simulink library "courseFollow_cl"  (R2018b)
settings: Solver=VariableStepAuto  StartTime=0.0  StopTime=10.0  RelTol=1e-3
values from neighbouring files (symbols this model uses):
  a = parseLogsout    [courseFollow_plant_ts.m]    (also in testUntilRoll_ts.m)
libraries: vectorNormalizer_ul x3, schmehlTangentRotation_ul x1, angleBtw2Vecs_ul x1
settings Model: Creator=James Reed  LastModifiedBy=jldanie5

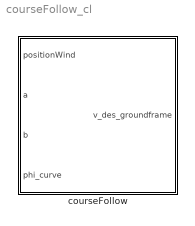
== system courseFollow_cl ==
  courseFollow : Subsystem

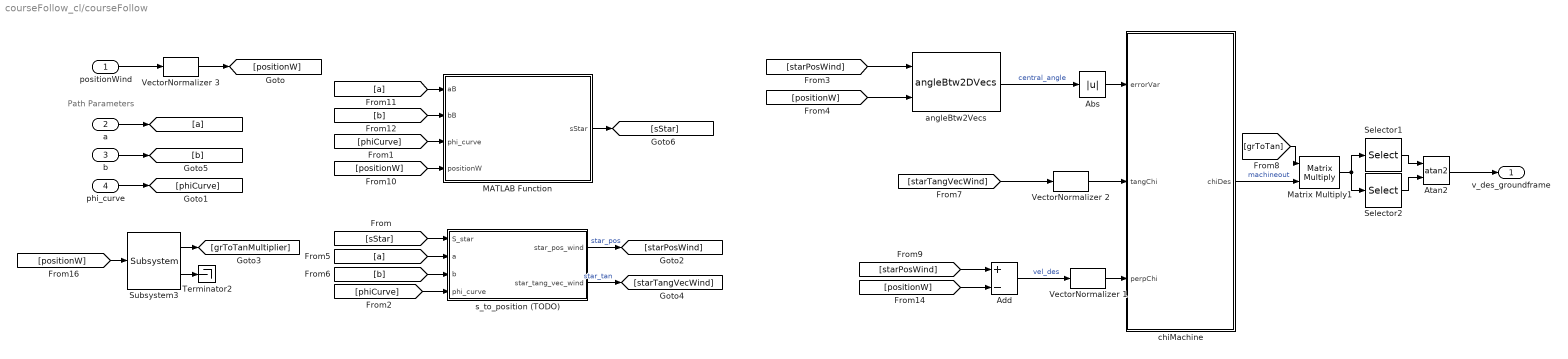
== system courseFollow_cl/courseFollow ==
  note: Path Parameters
  "positionWind " : Inport
  a : Inport  Port=2
  "b " : Inport  Port=3
  phi_curve : Inport  Port=4
  Abs : Abs
  Add : Sum  Inputs=+-
  Atan2 : Trigonometry  Operator=atan2
  MATLAB Function : MATLAB Function  TreatAsAtomicUnit=on
  Matrix Multiply1 : Product  Multiplication=Matrix(*)
  Selector1 : Selector  InputPortWidth=3  IndexOptions=Index vector (dialog)  Indices=2  OutputSizes=1
  Selector2 : Selector  InputPortWidth=3  IndexOptions=Index vector (dialog)  Indices=1  OutputSizes=1
  Subsystem3 : schmehlTangentRotation_ul/Subsystem  SystemSampleTime=-1
  Terminator2 : Terminator
  VectorNormalizer 1 : vectorNormalizer_ul/VectorNormalizer   SystemSampleTime=-1
  VectorNormalizer 2 : vectorNormalizer_ul/VectorNormalizer   SystemSampleTime=-1
  VectorNormalizer 3 : vectorNormalizer_ul/VectorNormalizer   SystemSampleTime=-1
  angleBtw2Vecs : angleBtw2Vecs_ul/angleBtw2DVecs  SystemSampleTime=-1
  chiMachine : Subsystem  mask{error_upper_lim=3*pi/180}
      mask prompts: error_upper_lim "Value of Error yielding 100% perpendicular"
  s_to_position (TODO) : Subsystem
  v_des_groundframe : Outport
  wires:
  VectorNormalizer 3/1 -> [positionW]
  [starPosWind] -> Add/1
  [phiCurve] -> MATLAB Function/3(phi_curve)
  [starPosWind] -> angleBtw2Vecs/1
  a/1 -> [a]
  VectorNormalizer 2/1 -> chiMachine/2(tangChi)
  chiMachine/1("chiDes ") -> Matrix Multiply1/2  "machineout"
  Add/1 -> VectorNormalizer 1/1  "vel_des"
  [positionW] -> MATLAB Function/4(positionW)
  phi_curve/1 -> [phiCurve]
  "b "/1 -> [b]
  [positionW] -> Subsystem3/1
  "positionWind "/1 -> VectorNormalizer 3/1
  [positionW] -> Add/2
  Subsystem3/1 -> [grToTanMultiplier]
  [b] -> s_to_position (TODO)/3(b)
  s_to_position (TODO)/1(star_pos_wind) -> [starPosWind]  "star_pos"
  [a] -> s_to_position (TODO)/2(a)
  VectorNormalizer 1/1 -> chiMachine/3("perpChi ")
  Abs/1 -> chiMachine/1("errorVar ")
  angleBtw2Vecs/1 -> Abs/1  "central_angle"
  [positionW] -> angleBtw2Vecs/2
  [b] -> MATLAB Function/2(bB)
  s_to_position (TODO)/2(star_tang_vec_wind) -> [starTangVecWind]  "star_tan"
  [sStar] -> s_to_position (TODO)/1(S_star)
  [starTangVecWind] -> VectorNormalizer 2/1
  MATLAB Function/1(sStar) -> [sStar]
  [a] -> MATLAB Function/1(aB)
  [phiCurve] -> s_to_position (TODO)/4(phi_curve)
  Subsystem3/2 -> Terminator2/1
  [grToTan] -> Matrix Multiply1/1
  Matrix Multiply1/1 -> Selector2/1, Selector1/1
  Selector1/1 -> Atan2/1
  Selector2/1 -> Atan2/2
  Atan2/1 -> v_des_groundframe/1

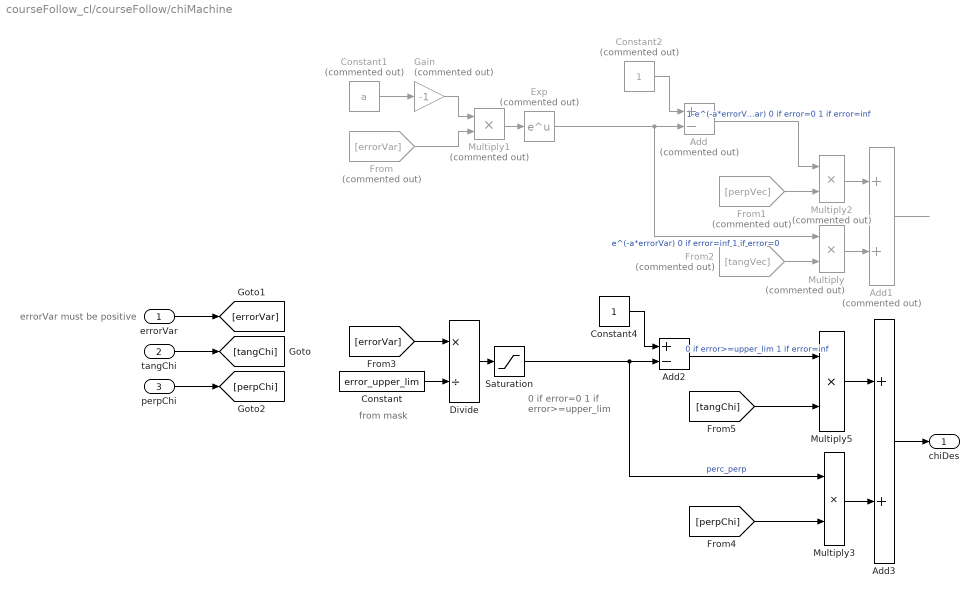
== system courseFollow_cl/courseFollow/chiMachine ==
  note: errorVar must be positive
  note: from mask
  note: 0 if error=0
      | 1 if error>=upper_lim
  "errorVar " : Inport
  tangChi : Inport  Port=2
  "perpChi " : Inport  Port=3
  Add : Sum  Commented=on  Inputs=+-
  Add1 : Sum  Commented=on
  Add2 : Sum  Inputs=+-
  Add3 : Sum
  Constant : Constant  Value=error_upper_lim
  Constant1 : Constant  Commented=on  Value=a
  Constant2 : Constant  Commented=on
  Constant4 : Constant
  Divide : Product  Inputs=*/
  Exp : Math  Commented=on  SaturateOnIntegerOverflow=on
  From : From  Commented=on  GotoTag=errorVar
  From1 : From  Commented=on  GotoTag=perpVec
  From2 : From  Commented=on  GotoTag=tangVec
  Gain : Gain  Commented=on  Gain=-1
  Multiply : Product  Commented=on
  Multiply1 : Product  Commented=on
  Multiply2 : Product  Commented=on
  Multiply3 : Product
  Multiply5 : Product
  Saturation : Saturate  UpperLimit=1  LowerLimit=0
  "chiDes " : Outport
  wires:
  [perpChi] -> Multiply3/2
  [tangChi] -> Multiply5/2
  Divide/1 -> Saturation/1
  Constant/1 -> Divide/2
  [errorVar] -> Divide/1
  Add2/1 -> Multiply5/1  "0 if error>=upper_lim 1 if error=inf"
  Multiply5/1 -> Add3/1
  Multiply3/1 -> Add3/2
  Add3/1 -> "chiDes "/1
  Saturation/1 -> Add2/2, Multiply3/1  "perc_perp"
  Constant4/1 -> Add2/1
  From2/1 -> Multiply/2
  From1/1 -> Multiply2/2
  Multiply/1 -> Add1/2
  Multiply2/1 -> Add1/1
  From/1 -> Multiply1/2
  "perpChi "/1 -> [perpChi]
  "errorVar "/1 -> [errorVar]
  Add1/1 -> ?
  Add/1 -> Multiply2/1  "1-e^(-a*errorVar) 0 if error=0 1 if error=inf"
  Constant2/1 -> Add/1
  Exp/1 -> Add/2, Multiply/1  "e^(-a*errorVar) 0 if error=inf 1 if error=0"
  Multiply1/1 -> Exp/1
  Gain/1 -> Multiply1/1
  Constant1/1 -> Gain/1
  tangChi/1 -> [tangChi]

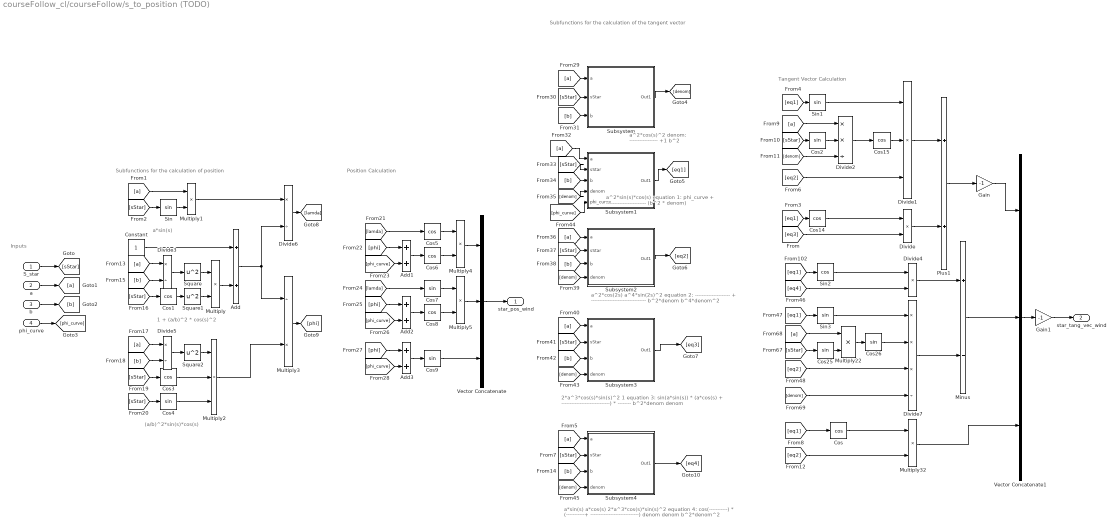
== system courseFollow_cl/courseFollow/s_to_position (TODO) ==
  note: (a/b)^2*sin(s)*cos(s)
  note: Subfunctions for the calculation of the tangent vector
  note: Position Calculation
  note: 1 + (a/b)^2 * cos(s)^2
  note: a^2*sin(s)*cos(s)
      | equation 1:   phi_curve + ------------------------
      | 					        (b^2 * denom)
  note: Tangent Vector Calculation
  note: a^2*cos(s)^2
      | denom: ----------------- +1
      |                      b^2
  note: a^2*cos(2s)                 a^4*sin(2s)^2
      | equation 2:   ---------------------  +  ---------------------------------
      |                          b^2*denom                 b^4*denom^2
  note: Inputs
  note: Subfunctions for the calculation of position
  note: a*sin(s)
  note: a*sin(s)       a*cos(s)   2*a^3*cos(s)*sin(s)^2
      | equation 4: cos(-----------) * (-----------+ -----------------------------)
      |                            denom        denom             b^2*denom^2
  note: 2*a^3*cos(s)*sin(s)^2         1
      | equation 3: sin(a*sin(s)) * (a*cos(s) + -----------------------------) * --------
      |                                                                      b^2*denom            denom
  S_star : Inport
  a : Inport  Port=2
  b : Inport  Port=3
  phi_curve : Inport  Port=4
  Add{,1..3} (4 alike) : Sum
  Constant : Constant
  Cos{,1,3,5..6,8,14..15} (8 alike) : Trigonometry  Operator=cos
  Cos{2,4,7,9,25..26} (6 alike) : Trigonometry
  Divide : Product  Inputs=**
  Divide1 : Product  Inputs=***
  Divide2 : Product  Inputs=**/
  Divide3 : Product  Inputs=*/
  Divide4 : Product  Inputs=**
  Divide5 : Product  Inputs=*/
  Divide6 : Product  Inputs=*/
  Divide7 : Product  Inputs=***/
  Gain : Gain  Gain=-1
  Gain1 : Gain  Gain=-1
  Minus : Sum  Inputs=+-
  Multiply{,1,4..5,22,32} (6 alike) : Product
  Multiply2 : Product  Inputs=3
  Multiply3 : Product  Inputs=/*
  Plus1 : Sum
  Sin : Trigonometry
  Sin1 : Trigonometry
  Sin2 : Trigonometry  Operator=cos
  Sin3 : Trigonometry
  Square : Math  Operator=square  SaturateOnIntegerOverflow=on
  Square1 : Math  Operator=square  SaturateOnIntegerOverflow=on
  Square2 : Math  Operator=square  SaturateOnIntegerOverflow=on
  Subsystem : Subsystem
  Subsystem1 : Subsystem
  Subsystem2 : Subsystem
  Subsystem3 : Subsystem
  Subsystem4 : Subsystem
  Vector Concatenate : Concatenate  NumInputs=3
  Vector Concatenate1 : Concatenate  NumInputs=3
  star_pos_wind : Outport
  star_tang_vec_wind : Outport  Port=2
  wires:
  Multiply4/1 -> Vector Concatenate/1
  [sStar] -> Subsystem/2(sStar)
  Cos25/1 -> Multiply22/2
  Cos6/1 -> Multiply4/2
  [eq1] -> Sin3/1
  [b] -> Subsystem1/3("b ")
  Subsystem3/1(Out1) -> [eq3]
  Divide1/1 -> Plus1/1
  [b] -> Subsystem2/3("b ")
  Cos5/1 -> Multiply4/1
  [phi] -> Add3/1
  [a] -> Subsystem2/1(a)
  Cos3/1 -> Multiply2/2
  [a] -> Subsystem3/1("a ")
  Cos8/1 -> Multiply5/2
  [sStar] -> Cos25/1
  [phi] -> Add1/1
  Multiply3/1 -> [phi]
  Square1/1 -> Multiply/2
  [sStar] -> Subsystem2/2(sStar)
  Add3/1 -> Cos9/1
  [eq2] -> Divide7/3
  [phi_curve] -> Add3/2
  Multiply2/1 -> Multiply3/2
  Plus1/1 -> Gain/1
  [sStar] -> Subsystem3/2("sStar ")
  Square/1 -> Multiply/1
  Subsystem4/1(Out1) -> [eq4]
  [sStar] -> Cos1/1
  Multiply22/1 -> Cos26/1
  Cos7/1 -> Multiply5/1
  Divide5/1 -> Square2/1
  [lamda] -> Cos7/1
  Add/1 -> Multiply3/1, Divide6/2
  [eq1] -> Sin2/1
  [denom] -> Subsystem2/4("denom ")
  [a] -> Divide3/1
  Divide/1 -> Plus1/2
  Cos26/1 -> Divide7/2
  Cos1/1 -> Square1/1
  [denom] -> Subsystem3/4("denom ")
  [b] -> Subsystem3/3("b ")
  Add2/1 -> Cos8/1
  [phi] -> Add2/1
  Divide3/1 -> Square/1
  [a] -> Subsystem1/1("a ")
  [sStar] -> Subsystem1/2("sStar ")
  [eq4] -> Divide4/2
  Divide4/1 -> Minus/1
  Divide6/1 -> [lamda]
  Sin2/1 -> Divide4/1
  [denom] -> Subsystem1/4(denom)
  Sin3/1 -> Divide7/1
  [a] -> Subsystem4/1("a ")
  Divide7/1 -> Minus/2
  [a] -> Multiply22/1
  [denom] -> Divide7/4
  Minus/1 -> Vector Concatenate1/2
  [sStar] -> Subsystem4/2("sStar ")
  Subsystem1/1(Out1) -> [eq1]
  [phi_curve] -> Subsystem1/5("phi_curve ")
  Cos15/1 -> Divide1/2
  [denom] -> Subsystem4/4("denom ")
  [b] -> Subsystem4/3("b ")
  [denom] -> Divide2/3
  [sStar] -> Cos2/1
  Cos2/1 -> Divide2/2
  [eq1] -> Cos14/1
  [eq1] -> Sin1/1
  Sin1/1 -> Divide1/1
  Cos14/1 -> Divide/1
  [eq2] -> Divide1/3
  [eq3] -> Divide/2
  [a] -> Divide2/1
  Divide2/1 -> Cos15/1
  b/1 -> [b]
  phi_curve/1 -> [phi_curve]
  Subsystem/1(Out1) -> [denom]
  Cos/1 -> Multiply32/1
  Multiply32/1 -> Vector Concatenate1/3
  Vector Concatenate1/1 -> Gain1/1
  [eq2] -> Multiply32/2
  Sin/1 -> Multiply1/2
  [a] -> Multiply1/1
  Vector Concatenate/1 -> star_pos_wind/1
  Gain/1 -> Vector Concatenate1/1
  Constant/1 -> Add/1
  Square2/1 -> Multiply2/1
  [sStar] -> Sin/1
  [b] -> Divide5/2
  [eq1] -> Cos/1
  [sStar] -> Cos3/1
  [sStar] -> Cos4/1
  [a] -> Divide5/1
  Multiply/1 -> Add/2
  Cos4/1 -> Multiply2/3
  Multiply1/1 -> Divide6/1
  [b] -> Divide3/2
  [lamda] -> Cos5/1
  [phi_curve] -> Add1/2
  Add1/1 -> Cos6/1
  [phi_curve] -> Add2/2
  Multiply5/1 -> Vector Concatenate/2
  Cos9/1 -> Vector Concatenate/3
  Subsystem2/1(Out1) -> [eq2]
  [a] -> Subsystem/1(a)
  S_star/1 -> [sStar]
  [b] -> Subsystem/3("b ")
  a/1 -> [a]
  Gain1/1 -> star_tang_vec_wind/1

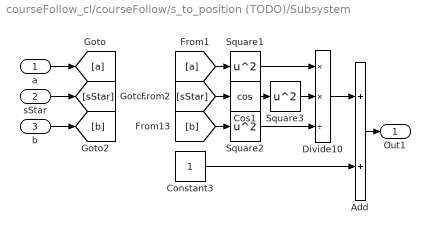
== system courseFollow_cl/courseFollow/s_to_position (TODO)/Subsystem ==
  a : Inport
  sStar : Inport  Port=2
  "b " : Inport  Port=3
  Add : Sum
  Constant3 : Constant
  Cos1 : Trigonometry  Operator=cos
  Divide10 : Product  Inputs=**/
  Square1 : Math  Operator=square  SaturateOnIntegerOverflow=on
  Square2 : Math  Operator=square  SaturateOnIntegerOverflow=on
  Square3 : Math  Operator=square  SaturateOnIntegerOverflow=on
  Out1 : Outport
  wires:
  Square3/1 -> Divide10/2
  Cos1/1 -> Square3/1
  "b "/1 -> [b]
  sStar/1 -> [sStar]
  a/1 -> [a]
  [b] -> Square2/1
  Square2/1 -> Divide10/3
  Divide10/1 -> Add/1
  [a] -> Square1/1
  Constant3/1 -> Add/2
  Square1/1 -> Divide10/1
  Add/1 -> Out1/1
  [sStar] -> Cos1/1

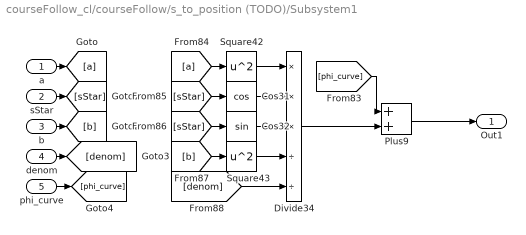
== system courseFollow_cl/courseFollow/s_to_position (TODO)/Subsystem1 ==
  "a " : Inport
  "sStar " : Inport  Port=2
  "b " : Inport  Port=3
  denom : Inport  Port=4
  "phi_curve " : Inport  Port=5
  Cos31 : Trigonometry  Operator=cos
  Cos32 : Trigonometry
  Divide34 : Product  Inputs=***//
  Plus9 : Sum
  Square42 : Math  Operator=square  SaturateOnIntegerOverflow=on
  Square43 : Math  Operator=square  SaturateOnIntegerOverflow=on
  Out1 : Outport
  wires:
  "phi_curve "/1 -> [phi_curve]
  "a "/1 -> [a]
  Cos32/1 -> Divide34/3
  Square43/1 -> Divide34/4
  [a] -> Square42/1
  Square42/1 -> Divide34/1
  [sStar] -> Cos31/1
  Plus9/1 -> Out1/1
  [denom] -> Divide34/5
  [sStar] -> Cos32/1
  Divide34/1 -> Plus9/2
  [b] -> Square43/1
  Cos31/1 -> Divide34/2
  "b "/1 -> [b]
  [phi_curve] -> Plus9/1
  "sStar "/1 -> [sStar]
  denom/1 -> [denom]

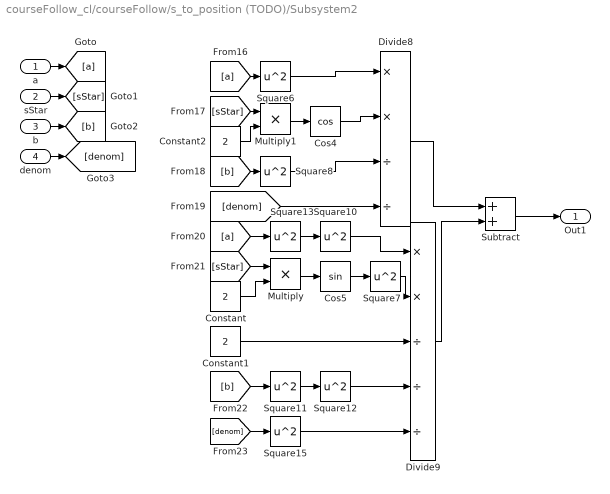
== system courseFollow_cl/courseFollow/s_to_position (TODO)/Subsystem2 ==
  a : Inport
  sStar : Inport  Port=2
  "b " : Inport  Port=3
  "denom " : Inport  Port=4
  Constant : Constant  Value=2
  Constant1 : Constant  Value=2
  Constant2 : Constant  Value=2
  Cos4 : Trigonometry  Operator=cos
  Cos5 : Trigonometry
  Divide8 : Product  Inputs=**//
  Divide9 : Product  Inputs=**///
  Multiply : Product
  Multiply1 : Product
  Square{6..8,10..13,15} (8 alike) : Math  Operator=square  SaturateOnIntegerOverflow=on
  Subtract : Sum
  Out1 : Outport
  wires:
  Constant2/1 -> Multiply1/2
  Multiply1/1 -> Cos4/1
  [sStar] -> Multiply1/1
  Constant1/1 -> Divide9/3
  Multiply/1 -> Cos5/1
  Constant/1 -> Multiply/2
  [denom] -> Divide8/4
  Square8/1 -> Divide8/3
  "denom "/1 -> [denom]
  "b "/1 -> [b]
  sStar/1 -> [sStar]
  a/1 -> [a]
  Divide9/1 -> Subtract/2
  Square7/1 -> Divide9/2
  Square15/1 -> Divide9/5
  Divide8/1 -> Subtract/1
  Cos5/1 -> Square7/1
  Subtract/1 -> Out1/1
  [sStar] -> Multiply/1
  Cos4/1 -> Divide8/2
  Square10/1 -> Divide9/1
  Square12/1 -> Divide9/4
  Square11/1 -> Square12/1
  [a] -> Square13/1
  [denom] -> Square15/1
  [a] -> Square6/1
  [b] -> Square8/1
  [b] -> Square11/1
  Square6/1 -> Divide8/1
  Square13/1 -> Square10/1

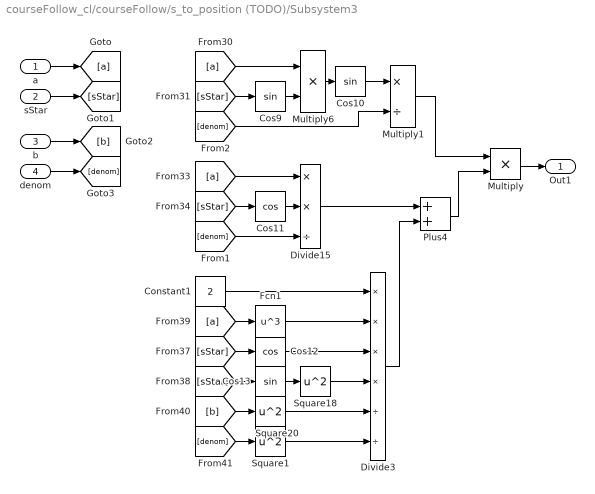
== system courseFollow_cl/courseFollow/s_to_position (TODO)/Subsystem3 ==
  "a " : Inport
  "sStar " : Inport  Port=2
  "b " : Inport  Port=3
  "denom " : Inport  Port=4
  Constant1 : Constant  Value=2
  Cos10 : Trigonometry
  Cos11 : Trigonometry  Operator=cos
  Cos12 : Trigonometry  Operator=cos
  Cos13 : Trigonometry
  Cos9 : Trigonometry
  Divide15 : Product  Inputs=**/
  Divide3 : Product  Inputs=****//
  Fcn1 : Fcn  Expr=u^3
  Multiply : Product
  Multiply1 : Product  Inputs=*/
  Multiply6 : Product
  Plus4 : Sum  Inputs=2
  Square1 : Math  Operator=square  SaturateOnIntegerOverflow=on
  Square18 : Math  Operator=square  SaturateOnIntegerOverflow=on
  Square20 : Math  Operator=square  SaturateOnIntegerOverflow=on
  Out1 : Outport
  wires:
  Multiply/1 -> Out1/1
  Multiply1/1 -> Multiply/1
  [denom] -> Multiply1/2
  Cos10/1 -> Multiply1/1
  [denom] -> Divide15/3
  Square1/1 -> Divide3/6
  [denom] -> Square1/1
  Cos12/1 -> Divide3/3
  [sStar] -> Cos12/1
  Divide15/1 -> Plus4/1
  Square18/1 -> Divide3/4
  Cos9/1 -> Multiply6/2
  Fcn1/1 -> Divide3/2
  Multiply6/1 -> Cos10/1
  Cos11/1 -> Divide15/2
  Square20/1 -> Divide3/5
  Constant1/1 -> Divide3/1
  [a] -> Fcn1/1
  Divide3/1 -> Plus4/2
  [sStar] -> Cos11/1
  Plus4/1 -> Multiply/2
  [a] -> Divide15/1
  [sStar] -> Cos13/1
  [sStar] -> Cos9/1
  [b] -> Square20/1
  Cos13/1 -> Square18/1
  [a] -> Multiply6/1
  "denom "/1 -> [denom]
  "b "/1 -> [b]
  "sStar "/1 -> [sStar]
  "a "/1 -> [a]

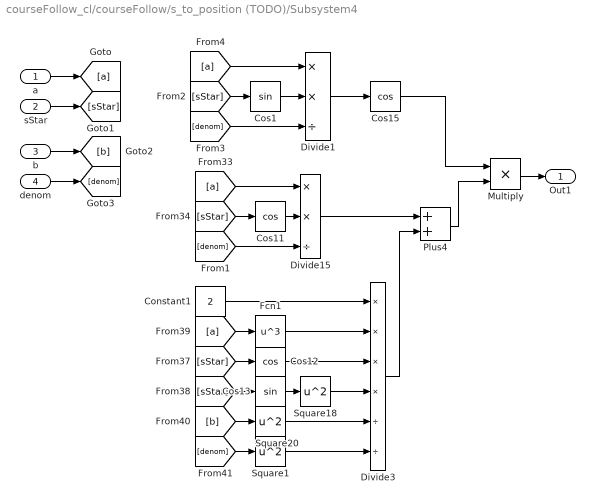
== system courseFollow_cl/courseFollow/s_to_position (TODO)/Subsystem4 ==
  "a " : Inport
  "sStar " : Inport  Port=2
  "b " : Inport  Port=3
  "denom " : Inport  Port=4
  Constant1 : Constant  Value=2
  Cos1 : Trigonometry
  Cos11 : Trigonometry  Operator=cos
  Cos12 : Trigonometry  Operator=cos
  Cos13 : Trigonometry
  Cos15 : Trigonometry  Operator=cos
  Divide1 : Product  Inputs=**/
  Divide15 : Product  Inputs=**/
  Divide3 : Product  Inputs=****//
  Fcn1 : Fcn  Expr=u^3
  Multiply : Product
  Plus4 : Sum  Inputs=2
  Square1 : Math  Operator=square  SaturateOnIntegerOverflow=on
  Square18 : Math  Operator=square  SaturateOnIntegerOverflow=on
  Square20 : Math  Operator=square  SaturateOnIntegerOverflow=on
  Out1 : Outport
  wires:
  Cos15/1 -> Multiply/1
  Divide1/1 -> Cos15/1
  [denom] -> Divide1/3
  Cos1/1 -> Divide1/2
  [a] -> Divide1/1
  [sStar] -> Cos1/1
  Multiply/1 -> Out1/1
  [denom] -> Divide15/3
  Square1/1 -> Divide3/6
  [denom] -> Square1/1
  Cos12/1 -> Divide3/3
  [sStar] -> Cos12/1
  Divide15/1 -> Plus4/1
  Square18/1 -> Divide3/4
  Fcn1/1 -> Divide3/2
  Cos11/1 -> Divide15/2
  Square20/1 -> Divide3/5
  Constant1/1 -> Divide3/1
  [a] -> Fcn1/1
  Divide3/1 -> Plus4/2
  [sStar] -> Cos11/1
  Plus4/1 -> Multiply/2
  [a] -> Divide15/1
  [sStar] -> Cos13/1
  [b] -> Square20/1
  Cos13/1 -> Square18/1
  "denom "/1 -> [denom]
  "b "/1 -> [b]
  "sStar "/1 -> [sStar]
  "a "/1 -> [a]

== matlab function courseFollow_cl/courseFollow/MATLAB Function ==
  data: aB input; sStar output; bB input; phi_curve input; positionW input
function sStar  = findClosestPoint(aB,bB,phi_curve,positionW)
%This functions purpose is to take the path and your current position and
%generate the location of the closest point in terms of the path parameter
%s
positionW=positionW';

%position in spherical cordinates 
[azP,elP,~] = cart2sph(positionW(1),positionW(2), positionW(3));

x0 = 0;
%the purpose of this function is to define a function the golden section
%method to minimize
lamda=@(s) aB*sin(s)/(1+(aB/bB)^2*cos(s)^2);
phi=@(s) (aB/bB)^2*sin(s)*cos(s)/(1 + (aB/bB)^2*cos(s)^2);
path = @(s)[cos(lamda(s)).*cos(phi_curve+phi(s));...
            sin(lamda(s)).*cos(phi_curve+phi(s));...
            sin(phi_curve+phi(s));];
centralAngle = @(s)acos(positionW*path(s)/(norm(path(s))*norm(positionW)));
      
% if the craft position has a greater elevation angle than the
% left right centerline of the path, and is on the right side of
% the path
if elP >=  phi_curve && azP  >=  0 %1st quadrant
   x0 = 0;

% if the craft position has a smaller elevation angle than the
% left right centerline of the path, and is on the right side of
% the path
elseif elP <= phi_curve && azP  >=  0 %4th quadrant
   x0 = (3*pi)/4;

   if elP <=  phi_curve && elP >= phi_curve-.08 && azP  >=  0 && azP <= .08 
       x0 = (5*pi)/4;
   end
% if the craft position has a greater elevation angle than the
% left right centerline of the path, and is on the left side of
% the path
elseif elP <= phi_curve && azP  <=  0 %3rd quadrant
   x0 = (7*pi)/4;

% if the craft position has a greater elevation angle than the
% left right centerline of the path, and is on the left side of
% the path
elseif elP >= phi_curve && azP  <=  0 %2nd quadrant
   x0 = (5*pi)/4;

end
           
          
%time in which the minimizer gives up if it has not found the closest point
StepTimeout = 1000;



StepSizeMultiplier = 2;
BoundingTimeout = 1000;

stepSize = .5;
xLeft = 0;
sign1 = 0;
MaxIterations = 1000;
%%%%%%%%%%%%%%%%%%%%%%%%%%%%%%%%%%%%%%%%%%%%%%%%%%%%%%%%%%%%%%%%%%%%%%%%%%%
%BOUNDING SECTION
%this section finds the bounds for the minimum to be located for faster
%searching
for tryCount = 1:StepTimeout
    % if f(<x0) is greater than f(x0) and f(x0) greater than f(>x0). 
    %negative sloping line
    if centralAngle(x0-stepSize) >= centralAngle(x0) && centralAngle(x0) >= centralAngle(x0+stepSize)
        sign1 = +1;
        break
        %  if f(<x0) is less than f(x0) and f(x0) less than f(>x0)
        %positive sloping line
    elseif  centralAngle(x0-stepSize) <= centralAngle(x0) &&...
            centralAngle(x0) <= centralAngle(x0+stepSize)
        sign1 = -1;
        break
    end
    stepSize = stepSize/2^tryCount;
end

xCurrent = x0;
for ii = 0:BoundingTimeout-1
    
    %the right bound = the current place *+(.5*2)^i
    xRight = xCurrent + sign1*stepSize*StepSizeMultiplier^ii;
    
    %if f(right bound) > f(current place) then stop 
    if centralAngle(xRight)>centralAngle(xCurrent)
        break
    end
    
    %replace your old left bound with the current guess at that iteration 
    xLeft = xCurrent;
    %new current place is your right bound
    xCurrent = xRight;
end
% if the curve is positive sloping between left and right bounds, sort 
if sign1 == -1
   xTemp  = sort([xLeft xRight]) ;
   xLeft  = xTemp(1);
   xRight= xTemp(2);
end

xl = xLeft;
xr = xRight;
%%%%%%%%%%%%%%%%%%%%%%%%%%%%%%%%%%%%%%%%%%%%%%%%%%%%%%%%%%%%%%%%%%%%%%%%%%%
% Begin golden section }
% this section finds the minimum central angle which is the closest point

tau = 1 - 0.38197;

for ii = 1:MaxIterations
    xTwo = (1-tau)*xl+tau*xr;
    xOne = tau*xl+(1-tau)*xr;
    fOne = centralAngle(xOne);
    fTwo = centralAngle(xTwo); 
    if fOne>fTwo %getting bigger 
        xl = xOne;
    end    
    if fOne<fTwo %&& xOne>sStarOld %getting smaller
        xr = xTwo;
    end
end

xLims = [xl xr];
if (xLims(1) + xLims(2))/2 >0
sStar = (xLims(1) + xLims(2))/2;

else 
sStar = ((xLims(1) + xLims(2))/2)+2*pi;   
end
end
